simulink model "attack_decay"  (R2020b)
settings: Solver=FixedStepAuto  StartTime=0.0  StopTime=stopTime  RelTol=1e-3
settings Model: Creator=t96f346  LastModifiedBy=tyler
settings DataIOCC: SaveOutput=off  SaveTime=off  ReturnWorkspaceOutputs=off
settings OptimizationCC: DefaultParameterBehavior=Inlined
settings ModelReferenceCC: EnableRefExpFcnMdlSchedulingChecks=off  ModelReferenceNumInstancesAllowed=Single

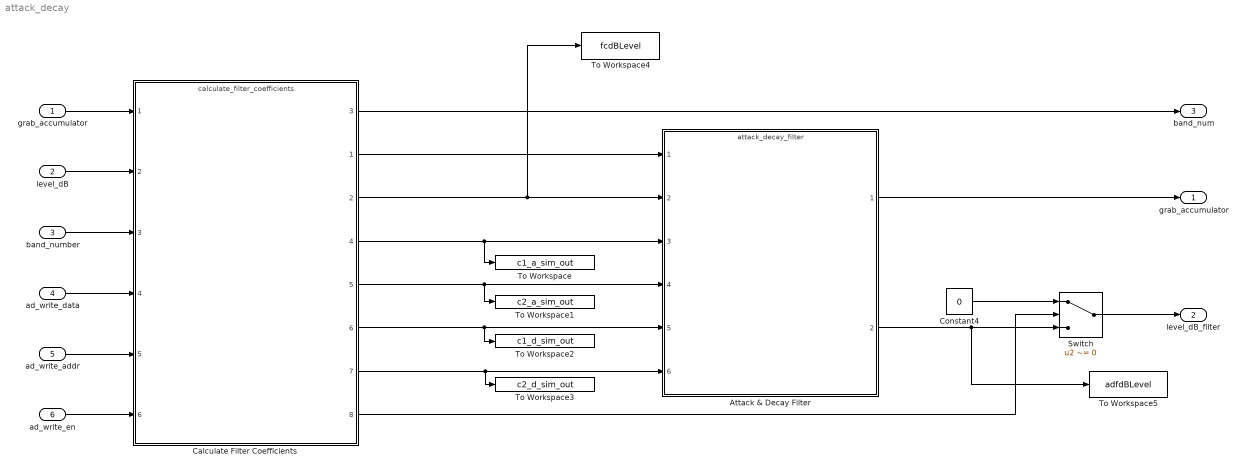
== system attack_decay ==
  grab_accumulator : Inport  OutDataTypeStr=boolean  PortDimensions=1
  level_dB : Inport  Port=2  OutDataTypeStr=input_type  PortDimensions=1
  band_number : Inport  Port=3  OutDataTypeStr=uint8  PortDimensions=1
  ad_write_data : Inport  Port=4  OutDataTypeStr=ad_coeff_type  PortDimensions=1
  ad_write_addr : Inport  Port=5  OutDataTypeStr=uint8  PortDimensions=1
  ad_write_en : Inport  Port=6  OutDataTypeStr=boolean  PortDimensions=1
  Attack & Decay Filter : ModelReference  ModelNameDialog=attack_decay_filter.slx  SimulationMode=Normal  ModelReferenceVersion=2.108
  Calculate Filter Coefficients : ModelReference  ModelNameDialog=calculate_filter_coefficients  SimulationMode=Normal  ModelReferenceVersion=2.70
      settings: PortSchema="{\"entries\":[{\"content\":{\"sides\":[{\"content\":{\"connectorIds\":[\"In1\",\"In2\",\"In3\",\"In4\",\"In5\",\"In6\"]},\"type\":\"ConnectorPlacement.EquallySpacedRectSide\",\"uuid\":\"e16ade1d-f377-4672-8f05-fbcc74c5c629\"},{\"content\":{\"connectorIds\":[\"Out3\",\"Out1\",\"Out2\",\"Out4\",\"Out5\",\"Out6\",\"Out7\",\"Out8\"],\"side\":\"RIGHT\"},\"type\":\"ConnectorPlacement.EquallySpacedRectSide\",\"uuid\":\"6cc420d8-b618-4c12-be31-c4666e1f7b82\"},{\"content\":{\"connectorIds\":[],\"side\":\"TOP\"},\"type\":\"ConnectorPlacement.EquallySpacedRectSide\",\"uuid\":\"0b0e1b93-5f65-46b5-81b0-f9e508c8aec7\"},{\"content\":{\"connectorIds\":[],\"side\":\"HIDDEN\"},\"type\":\"ConnectorPlacement.EquallySpacedRectSide\",\"uuid\":\"caaf3158-30dd-4639-b718-0824916c80e1\"}]},\"type\":\"ConnectorPlacement.EquallySpacedConnector\",\"uuid\":\"27f558c7-8c94-4b0c-b056-fbd050fb838e\"}],\"packageUris\":[\"http://schema.mathworks.com/mf0/Connector/R2020b\"],\"version\":\"1.0\"}"
      mask Display: disp(sprintf(['Programmable Look-Up Table\nMemory Used: %d bits, Address Width: %d\n' tableFnParam ': %.2d <= x <= %.2d\n Maximum Error: %.2d %%'], 2*2^RAM_SIZE*W_bits, RAM_SIZE, minVal, maxVal, 100*maxErr)); port_label('input',1,'Data_In'); port_label('input',2,'Table_Wr_Data'); port_label('input',3,'Table_RW_Addr'); port_label('input',4,'Table_Wr_En'); port_label('output',1,'Data_Out'); port_label('output',2,'Table_RW_Dout');
  Constant4 : Constant  Value=0  OutDataTypeStr=Inherit: Inherit via back propagation  SampleTime=-1
  Switch : Switch  Criteria=u2 ~= 0  OutDataTypeStr=Inherit: Inherit via back propagation
  To Workspace : ToWorkspace  VariableName=c1_a_sim_out  SampleTime=-1
  To Workspace1 : ToWorkspace  VariableName=c2_a_sim_out  SampleTime=-1
  To Workspace2 : ToWorkspace  VariableName=c1_d_sim_out  SampleTime=-1
  To Workspace3 : ToWorkspace  VariableName=c2_d_sim_out  SampleTime=-1
  To Workspace4 : ToWorkspace  VariableName=fcdBLevel  SaveFormat=Timeseries  SampleTime=-1
  To Workspace5 : ToWorkspace  VariableName=adfdBLevel  SaveFormat=Timeseries  SampleTime=-1
  "grab_accumulator " : Outport  PortDimensions=1
  level_dB_filter : Outport  Port=2  PortDimensions=[1 1]
  "band_num " : Outport  Port=3  PortDimensions=1
  wires:
  grab_accumulator/1 -> Calculate Filter Coefficients/1
  Calculate Filter Coefficients/7 -> Attack & Decay Filter/6, To Workspace3/1
  Calculate Filter Coefficients/6 -> Attack & Decay Filter/5, To Workspace2/1
  Calculate Filter Coefficients/5 -> Attack & Decay Filter/4, To Workspace1/1
  Calculate Filter Coefficients/4 -> Attack & Decay Filter/3, To Workspace/1
  Constant4/1 -> Switch/1
  ad_write_en/1 -> Calculate Filter Coefficients/6
  ad_write_addr/1 -> Calculate Filter Coefficients/5
  ad_write_data/1 -> Calculate Filter Coefficients/4
  band_number/1 -> Calculate Filter Coefficients/3
  level_dB/1 -> Calculate Filter Coefficients/2
  Switch/1 -> level_dB_filter/1
  Attack & Decay Filter/1 -> "grab_accumulator "/1
  Attack & Decay Filter/2 -> To Workspace5/1, Switch/3
  Calculate Filter Coefficients/2 -> Attack & Decay Filter/2, To Workspace4/1
  Calculate Filter Coefficients/1 -> Attack & Decay Filter/1
  Calculate Filter Coefficients/3 -> "band_num "/1
  Calculate Filter Coefficients/8 -> Switch/2
